simulink model "Model_with_decision_and_sieve"  (R2022a)
settings: Solver=VariableStepAuto  StartTime=0.0  StopTime=1000000  RelTol=1e-3
undefined symbols (not defined in the file): Coefficient_value, Enable_X, Enable_Y, N, s1, s10, s11, s12, s13, s14, s15, s16, s17, s18, s19, s2, s20, s21, s22, s23, s24, s25, s26, s27, s28, s29, s3, s30, s4, s5, s6, s7, s8, s9
libraries: simulink x37, dspsigops x2
(part 4 of 5)

== system Model_with_decision_and_sieve/Y12 ==
  Y1 : Inport  OutDataTypeStr=fixdt(0,1,0)  LockScale=on
  Y2 : Inport  Port=2  OutDataTypeStr=fixdt(0,1,0)  LockScale=on
  Y3 : Inport  Port=3  OutDataTypeStr=fixdt(0,1,0)  LockScale=on
  Y4 : Inport  Port=4  OutDataTypeStr=fixdt(0,1,0)  LockScale=on
  Y5 : Inport  Port=5  OutDataTypeStr=fixdt(0,1,0)  LockScale=on
  Y6 : Inport  Port=6  OutDataTypeStr=fixdt(0,1,0)  LockScale=on
  Y7 : Inport  Port=7  OutDataTypeStr=fixdt(0,1,0)  LockScale=on
  Y8 : Inport  Port=8  OutDataTypeStr=fixdt(0,1,0)  LockScale=on
  Y9 : Inport  Port=9  OutDataTypeStr=fixdt(0,1,0)  LockScale=on
  Y10 : Inport  Port=10  OutDataTypeStr=fixdt(0,1,0)  LockScale=on
  Y11 : Inport  Port=11  OutDataTypeStr=fixdt(0,1,0)  LockScale=on
  Y12 : Inport  Port=12  OutDataTypeStr=fixdt(0,1,0)  LockScale=on
  Y13 : Inport  Port=13  OutDataTypeStr=fixdt(0,1,0)  LockScale=on
  Y14 : Inport  Port=14  OutDataTypeStr=fixdt(0,1,0)  LockScale=on
  Y15 : Inport  Port=15  OutDataTypeStr=fixdt(0,1,0)  LockScale=on
  X : Inport  Port=16
  N : Inport  Port=17  LockScale=on
  shifted_coeff : Inport  Port=18  LockScale=on
  EN_Y : Inport  Port=19  OutDataTypeStr=fixdt(0,1,0)  LockScale=on
  Add : Sum  Inputs=++++++++++++++++
  Add2 : Sum  Inputs=+-
  Constant : Constant  Value=2
  Constant1 : Constant  Value=4
  Constant15 : Constant  Value=128
  Constant16 : Constant  Value=256
  Constant17 : Constant  Value=512
  Constant18 : Constant  Value=1024
  Constant19 : Constant  Value=2048
  Constant2 : Constant  Value=8
  Constant20 : Constant  Value=4096
  Constant21 : Constant  Value=8192
  Constant22 : Constant  Value=16384
  Constant3 : Constant  Value=16
  Constant34 : Constant  Value=32768
  Constant4 : Constant  Value=32
  Constant6 : Constant
  Constant8 : Constant  Value=64
  NOT : Logic  Operator=NOT  IconShape=distinctive  AllPortsSameDT=off  OutDataTypeStr=boolean
  Product{,1..6,8,16..23,35,142} (18 alike) : Product
  Switch_2 : Switch  Criteria=u2 ~= 0  OutDataTypeStr=fixdt(0,1,0)  SaturateOnIntegerOverflow=off  InputSameDT=off
  E_Y : Outport  LockScale=on
  wires:
  Constant/1 -> Product/2
  Y1/1 -> Product/1
  Constant1/1 -> Product1/2
  Y2/1 -> Product1/1
  Constant2/1 -> Product2/2
  Y3/1 -> Product2/1
  Constant6/1 -> Add/1
  Product/1 -> Add/2
  Product1/1 -> Add/3
  Product2/1 -> Add/4
  Add/1 -> Product6/1
  Add2/1 -> Product8/2, Product8/1
  Product4/1 -> Add/6
  Constant4/1 -> Product4/2
  Constant8/1 -> Product5/2
  Y6/1 -> Product5/1
  Product3/1 -> Add/5
  Y4/1 -> Product3/1
  Product5/1 -> Add/7
  Y5/1 -> Product4/1
  Constant3/1 -> Product3/2
  Product19/1 -> Add/11
  Constant20/1 -> Product21/2
  Constant18/1 -> Product19/2
  Product18/1 -> Add/10
  Constant15/1 -> Product16/2
  Constant16/1 -> Product17/2
  Y11/1 -> Product20/1
  Product20/1 -> Add/12
  Y8/1 -> Product17/1
  Y10/1 -> Product19/1
  Y7/1 -> Product16/1
  Constant19/1 -> Product20/2
  Product16/1 -> Add/8
  Y9/1 -> Product18/1
  Constant17/1 -> Product18/2
  Product21/1 -> Add/13
  Switch_2/1 -> Product21/1
  Product17/1 -> Add/9
  Y14/1 -> Product23/1
  Product22/1 -> Add/14
  Product23/1 -> Add/15
  Constant21/1 -> Product22/2
  Constant22/1 -> Product23/2
  [EN_Y] -> Switch_2/2
  Y12/1 -> Switch_2/3, NOT/1  "PBIT28"
  NOT/1 -> Switch_2/1
  Y13/1 -> Product22/1
  EN_Y/1 -> [EN_Y]
  shifted_coeff/1 -> [shifted_coeff]
  Product142/1 -> E_Y/1
  [shifted_coeff] -> Product142/2
  Product6/1 -> Add2/1
  Product8/1 -> Product142/1
  N/1 -> Add2/2
  X/1 -> Product6/2
  Y15/1 -> Product35/1
  Product35/1 -> Add/16
  Constant34/1 -> Product35/2

== system Model_with_decision_and_sieve/Y13 ==
  Y1 : Inport  OutDataTypeStr=fixdt(0,1,0)  LockScale=on
  Y2 : Inport  Port=2  OutDataTypeStr=fixdt(0,1,0)  LockScale=on
  Y3 : Inport  Port=3  OutDataTypeStr=fixdt(0,1,0)  LockScale=on
  Y4 : Inport  Port=4  OutDataTypeStr=fixdt(0,1,0)  LockScale=on
  Y5 : Inport  Port=5  OutDataTypeStr=fixdt(0,1,0)  LockScale=on
  Y6 : Inport  Port=6  OutDataTypeStr=fixdt(0,1,0)  LockScale=on
  Y7 : Inport  Port=7  OutDataTypeStr=fixdt(0,1,0)  LockScale=on
  Y8 : Inport  Port=8  OutDataTypeStr=fixdt(0,1,0)  LockScale=on
  Y9 : Inport  Port=9  OutDataTypeStr=fixdt(0,1,0)  LockScale=on
  Y10 : Inport  Port=10  OutDataTypeStr=fixdt(0,1,0)  LockScale=on
  Y11 : Inport  Port=11  OutDataTypeStr=fixdt(0,1,0)  LockScale=on
  Y12 : Inport  Port=12  OutDataTypeStr=fixdt(0,1,0)  LockScale=on
  Y13 : Inport  Port=13  OutDataTypeStr=fixdt(0,1,0)  LockScale=on
  Y14 : Inport  Port=14  OutDataTypeStr=fixdt(0,1,0)  LockScale=on
  Y15 : Inport  Port=15  OutDataTypeStr=fixdt(0,1,0)  LockScale=on
  X : Inport  Port=16
  N : Inport  Port=17  LockScale=on
  shifted_coeff : Inport  Port=18  LockScale=on
  EN_Y : Inport  Port=19  OutDataTypeStr=fixdt(0,1,0)  LockScale=on
  Add : Sum  Inputs=++++++++++++++++
  Add2 : Sum  Inputs=+-
  Constant : Constant  Value=2
  Constant1 : Constant  Value=4
  Constant15 : Constant  Value=128
  Constant16 : Constant  Value=256
  Constant17 : Constant  Value=512
  Constant18 : Constant  Value=1024
  Constant19 : Constant  Value=2048
  Constant2 : Constant  Value=8
  Constant20 : Constant  Value=4096
  Constant21 : Constant  Value=8192
  Constant22 : Constant  Value=16384
  Constant3 : Constant  Value=16
  Constant34 : Constant  Value=32768
  Constant4 : Constant  Value=32
  Constant6 : Constant
  Constant8 : Constant  Value=64
  NOT : Logic  Operator=NOT  IconShape=distinctive  AllPortsSameDT=off  OutDataTypeStr=boolean
  Product{,1..6,8,16..23,35,142} (18 alike) : Product
  Switch_2 : Switch  Criteria=u2 ~= 0  OutDataTypeStr=fixdt(0,1,0)  SaturateOnIntegerOverflow=off  InputSameDT=off
  E_Y : Outport  LockScale=on
  wires:
  Constant34/1 -> Product35/2
  Product35/1 -> Add/16
  Y15/1 -> Product35/1
  X/1 -> Product6/2
  N/1 -> Add2/2
  Product8/1 -> Product142/1
  Product6/1 -> Add2/1
  [shifted_coeff] -> Product142/2
  Product142/1 -> E_Y/1
  shifted_coeff/1 -> [shifted_coeff]
  EN_Y/1 -> [EN_Y]
  Switch_2/1 -> Product22/1
  NOT/1 -> Switch_2/1
  Y13/1 -> Switch_2/3, NOT/1  "PBIT28"
  [EN_Y] -> Switch_2/2
  Constant22/1 -> Product23/2
  Constant21/1 -> Product22/2
  Product23/1 -> Add/15
  Product22/1 -> Add/14
  Y14/1 -> Product23/1
  Product17/1 -> Add/9
  Y12/1 -> Product21/1
  Product21/1 -> Add/13
  Constant17/1 -> Product18/2
  Y9/1 -> Product18/1
  Product16/1 -> Add/8
  Constant19/1 -> Product20/2
  Y7/1 -> Product16/1
  Y10/1 -> Product19/1
  Y8/1 -> Product17/1
  Product20/1 -> Add/12
  Y11/1 -> Product20/1
  Constant16/1 -> Product17/2
  Constant15/1 -> Product16/2
  Product18/1 -> Add/10
  Constant18/1 -> Product19/2
  Constant20/1 -> Product21/2
  Product19/1 -> Add/11
  Constant3/1 -> Product3/2
  Y5/1 -> Product4/1
  Product5/1 -> Add/7
  Y4/1 -> Product3/1
  Product3/1 -> Add/5
  Y6/1 -> Product5/1
  Constant8/1 -> Product5/2
  Constant4/1 -> Product4/2
  Product4/1 -> Add/6
  Add2/1 -> Product8/1, Product8/2
  Add/1 -> Product6/1
  Product2/1 -> Add/4
  Product1/1 -> Add/3
  Product/1 -> Add/2
  Constant6/1 -> Add/1
  Y3/1 -> Product2/1
  Constant2/1 -> Product2/2
  Y2/1 -> Product1/1
  Constant1/1 -> Product1/2
  Y1/1 -> Product/1
  Constant/1 -> Product/2

== system Model_with_decision_and_sieve/Y14 ==
  Y1 : Inport  OutDataTypeStr=fixdt(0,1,0)  LockScale=on
  Y2 : Inport  Port=2  OutDataTypeStr=fixdt(0,1,0)  LockScale=on
  Y3 : Inport  Port=3  OutDataTypeStr=fixdt(0,1,0)  LockScale=on
  Y4 : Inport  Port=4  OutDataTypeStr=fixdt(0,1,0)  LockScale=on
  Y5 : Inport  Port=5  OutDataTypeStr=fixdt(0,1,0)  LockScale=on
  Y6 : Inport  Port=6  OutDataTypeStr=fixdt(0,1,0)  LockScale=on
  Y7 : Inport  Port=7  OutDataTypeStr=fixdt(0,1,0)  LockScale=on
  Y8 : Inport  Port=8  OutDataTypeStr=fixdt(0,1,0)  LockScale=on
  Y9 : Inport  Port=9  OutDataTypeStr=fixdt(0,1,0)  LockScale=on
  Y10 : Inport  Port=10  OutDataTypeStr=fixdt(0,1,0)  LockScale=on
  Y11 : Inport  Port=11  OutDataTypeStr=fixdt(0,1,0)  LockScale=on
  Y12 : Inport  Port=12  OutDataTypeStr=fixdt(0,1,0)  LockScale=on
  Y13 : Inport  Port=13  OutDataTypeStr=fixdt(0,1,0)  LockScale=on
  Y14 : Inport  Port=14  OutDataTypeStr=fixdt(0,1,0)  LockScale=on
  Y15 : Inport  Port=15  OutDataTypeStr=fixdt(0,1,0)  LockScale=on
  X : Inport  Port=16
  N : Inport  Port=17  LockScale=on
  shifted_coeff : Inport  Port=18  LockScale=on
  EN_Y : Inport  Port=19  OutDataTypeStr=fixdt(0,1,0)  LockScale=on
  Add : Sum  Inputs=++++++++++++++++
  Add2 : Sum  Inputs=+-
  Constant : Constant  Value=2
  Constant1 : Constant  Value=4
  Constant15 : Constant  Value=128
  Constant16 : Constant  Value=256
  Constant17 : Constant  Value=512
  Constant18 : Constant  Value=1024
  Constant19 : Constant  Value=2048
  Constant2 : Constant  Value=8
  Constant20 : Constant  Value=4096
  Constant21 : Constant  Value=8192
  Constant22 : Constant  Value=16384
  Constant3 : Constant  Value=16
  Constant34 : Constant  Value=32768
  Constant4 : Constant  Value=32
  Constant6 : Constant
  Constant8 : Constant  Value=64
  NOT : Logic  Operator=NOT  IconShape=distinctive  AllPortsSameDT=off  OutDataTypeStr=boolean
  Product{,1..6,8,16..23,35,142} (18 alike) : Product
  Switch_2 : Switch  Criteria=u2 ~= 0  OutDataTypeStr=fixdt(0,1,0)  SaturateOnIntegerOverflow=off  InputSameDT=off
  E_Y : Outport  LockScale=on
  wires:
  Constant/1 -> Product/2
  Y1/1 -> Product/1
  Constant1/1 -> Product1/2
  Y2/1 -> Product1/1
  Constant2/1 -> Product2/2
  Y3/1 -> Product2/1
  Constant6/1 -> Add/1
  Product/1 -> Add/2
  Product1/1 -> Add/3
  Product2/1 -> Add/4
  Add/1 -> Product6/1
  Add2/1 -> Product8/2, Product8/1
  Product4/1 -> Add/6
  Constant4/1 -> Product4/2
  Constant8/1 -> Product5/2
  Y6/1 -> Product5/1
  Product3/1 -> Add/5
  Y4/1 -> Product3/1
  Product5/1 -> Add/7
  Y5/1 -> Product4/1
  Constant3/1 -> Product3/2
  Product19/1 -> Add/11
  Constant20/1 -> Product21/2
  Constant18/1 -> Product19/2
  Product18/1 -> Add/10
  Constant15/1 -> Product16/2
  Constant16/1 -> Product17/2
  Y11/1 -> Product20/1
  Product20/1 -> Add/12
  Y8/1 -> Product17/1
  Y10/1 -> Product19/1
  Y7/1 -> Product16/1
  Constant19/1 -> Product20/2
  Product16/1 -> Add/8
  Y9/1 -> Product18/1
  Constant17/1 -> Product18/2
  Product21/1 -> Add/13
  Y12/1 -> Product21/1
  Product17/1 -> Add/9
  Switch_2/1 -> Product23/1
  Product22/1 -> Add/14
  Product23/1 -> Add/15
  Constant21/1 -> Product22/2
  Constant22/1 -> Product23/2
  [EN_Y] -> Switch_2/2
  Y14/1 -> Switch_2/3, NOT/1  "PBIT28"
  NOT/1 -> Switch_2/1
  Y13/1 -> Product22/1
  EN_Y/1 -> [EN_Y]
  shifted_coeff/1 -> [shifted_coeff]
  Product142/1 -> E_Y/1
  [shifted_coeff] -> Product142/2
  Product6/1 -> Add2/1
  Product8/1 -> Product142/1
  N/1 -> Add2/2
  X/1 -> Product6/2
  Y15/1 -> Product35/1
  Product35/1 -> Add/16
  Constant34/1 -> Product35/2

== system Model_with_decision_and_sieve/Y15 ==
  Y1 : Inport  OutDataTypeStr=fixdt(0,1,0)  LockScale=on
  Y2 : Inport  Port=2  OutDataTypeStr=fixdt(0,1,0)  LockScale=on
  Y3 : Inport  Port=3  OutDataTypeStr=fixdt(0,1,0)  LockScale=on
  Y4 : Inport  Port=4  OutDataTypeStr=fixdt(0,1,0)  LockScale=on
  Y5 : Inport  Port=5  OutDataTypeStr=fixdt(0,1,0)  LockScale=on
  Y6 : Inport  Port=6  OutDataTypeStr=fixdt(0,1,0)  LockScale=on
  Y7 : Inport  Port=7  OutDataTypeStr=fixdt(0,1,0)  LockScale=on
  Y8 : Inport  Port=8  OutDataTypeStr=fixdt(0,1,0)  LockScale=on
  Y9 : Inport  Port=9  OutDataTypeStr=fixdt(0,1,0)  LockScale=on
  Y10 : Inport  Port=10  OutDataTypeStr=fixdt(0,1,0)  LockScale=on
  Y11 : Inport  Port=11  OutDataTypeStr=fixdt(0,1,0)  LockScale=on
  Y12 : Inport  Port=12  OutDataTypeStr=fixdt(0,1,0)  LockScale=on
  Y13 : Inport  Port=13  OutDataTypeStr=fixdt(0,1,0)  LockScale=on
  Y14 : Inport  Port=14  OutDataTypeStr=fixdt(0,1,0)  LockScale=on
  Y15 : Inport  Port=15  OutDataTypeStr=fixdt(0,1,0)  LockScale=on
  X : Inport  Port=16
  N : Inport  Port=17  LockScale=on
  shifted_coeff : Inport  Port=18  LockScale=on
  EN_Y : Inport  Port=19  OutDataTypeStr=fixdt(0,1,0)  LockScale=on
  Add : Sum  Inputs=++++++++++++++++
  Add2 : Sum  Inputs=+-
  Constant : Constant  Value=2
  Constant1 : Constant  Value=4
  Constant15 : Constant  Value=128
  Constant16 : Constant  Value=256
  Constant17 : Constant  Value=512
  Constant18 : Constant  Value=1024
  Constant19 : Constant  Value=2048
  Constant2 : Constant  Value=8
  Constant20 : Constant  Value=4096
  Constant21 : Constant  Value=8192
  Constant22 : Constant  Value=16384
  Constant3 : Constant  Value=16
  Constant34 : Constant  Value=32768
  Constant4 : Constant  Value=32
  Constant6 : Constant
  Constant8 : Constant  Value=64
  NOT : Logic  Operator=NOT  IconShape=distinctive  AllPortsSameDT=off  OutDataTypeStr=boolean
  Product{,1..6,8,16..23,35,142} (18 alike) : Product
  Switch_2 : Switch  Criteria=u2 ~= 0  OutDataTypeStr=fixdt(0,1,0)  SaturateOnIntegerOverflow=off  InputSameDT=off
  E_Y : Outport  LockScale=on
  wires:
  Constant34/1 -> Product35/2
  Product35/1 -> Add/16
  Switch_2/1 -> Product35/1
  X/1 -> Product6/2
  N/1 -> Add2/2
  Product8/1 -> Product142/1
  Product6/1 -> Add2/1
  [shifted_coeff] -> Product142/2
  Product142/1 -> E_Y/1
  shifted_coeff/1 -> [shifted_coeff]
  EN_Y/1 -> [EN_Y]
  Y13/1 -> Product22/1
  NOT/1 -> Switch_2/1
  Y15/1 -> NOT/1, Switch_2/3  "PBIT28"
  [EN_Y] -> Switch_2/2
  Constant22/1 -> Product23/2
  Constant21/1 -> Product22/2
  Product23/1 -> Add/15
  Product22/1 -> Add/14
  Y14/1 -> Product23/1
  Product17/1 -> Add/9
  Y12/1 -> Product21/1
  Product21/1 -> Add/13
  Constant17/1 -> Product18/2
  Y9/1 -> Product18/1
  Product16/1 -> Add/8
  Constant19/1 -> Product20/2
  Y7/1 -> Product16/1
  Y10/1 -> Product19/1
  Y8/1 -> Product17/1
  Product20/1 -> Add/12
  Y11/1 -> Product20/1
  Constant16/1 -> Product17/2
  Constant15/1 -> Product16/2
  Product18/1 -> Add/10
  Constant18/1 -> Product19/2
  Constant20/1 -> Product21/2
  Product19/1 -> Add/11
  Constant3/1 -> Product3/2
  Y5/1 -> Product4/1
  Product5/1 -> Add/7
  Y4/1 -> Product3/1
  Product3/1 -> Add/5
  Y6/1 -> Product5/1
  Constant8/1 -> Product5/2
  Constant4/1 -> Product4/2
  Product4/1 -> Add/6
  Add2/1 -> Product8/1, Product8/2
  Add/1 -> Product6/1
  Product2/1 -> Add/4
  Product1/1 -> Add/3
  Product/1 -> Add/2
  Constant6/1 -> Add/1
  Y3/1 -> Product2/1
  Constant2/1 -> Product2/2
  Y2/1 -> Product1/1
  Constant1/1 -> Product1/2
  Y1/1 -> Product/1
  Constant/1 -> Product/2

== system Model_with_decision_and_sieve/Y2 ==
  Y1 : Inport  OutDataTypeStr=fixdt(0,1,0)  LockScale=on
  Y2 : Inport  Port=2  OutDataTypeStr=fixdt(0,1,0)  LockScale=on
  Y3 : Inport  Port=3  OutDataTypeStr=fixdt(0,1,0)  LockScale=on
  Y4 : Inport  Port=4  OutDataTypeStr=fixdt(0,1,0)  LockScale=on
  Y5 : Inport  Port=5  OutDataTypeStr=fixdt(0,1,0)  LockScale=on
  Y6 : Inport  Port=6  OutDataTypeStr=fixdt(0,1,0)  LockScale=on
  Y7 : Inport  Port=7  OutDataTypeStr=fixdt(0,1,0)  LockScale=on
  Y8 : Inport  Port=8  OutDataTypeStr=fixdt(0,1,0)  LockScale=on
  Y9 : Inport  Port=9  OutDataTypeStr=fixdt(0,1,0)  LockScale=on
  Y10 : Inport  Port=10  OutDataTypeStr=fixdt(0,1,0)  LockScale=on
  Y11 : Inport  Port=11  OutDataTypeStr=fixdt(0,1,0)  LockScale=on
  Y12 : Inport  Port=12  OutDataTypeStr=fixdt(0,1,0)  LockScale=on
  Y13 : Inport  Port=13  OutDataTypeStr=fixdt(0,1,0)  LockScale=on
  Y14 : Inport  Port=14  OutDataTypeStr=fixdt(0,1,0)  LockScale=on
  Y15 : Inport  Port=15  OutDataTypeStr=fixdt(0,1,0)  LockScale=on
  X : Inport  Port=16
  N : Inport  Port=17  LockScale=on
  shifted_coeff : Inport  Port=18  LockScale=on
  EN_Y : Inport  Port=19  OutDataTypeStr=fixdt(0,1,0)  LockScale=on
  Add : Sum  Inputs=++++++++++++++++
  Add2 : Sum  Inputs=+-
  Constant : Constant  Value=2
  Constant1 : Constant  Value=4
  Constant15 : Constant  Value=128
  Constant16 : Constant  Value=256
  Constant17 : Constant  Value=512
  Constant18 : Constant  Value=1024
  Constant19 : Constant  Value=2048
  Constant2 : Constant  Value=8
  Constant20 : Constant  Value=4096
  Constant21 : Constant  Value=8192
  Constant22 : Constant  Value=16384
  Constant3 : Constant  Value=16
  Constant34 : Constant  Value=32768
  Constant4 : Constant  Value=32
  Constant6 : Constant
  Constant8 : Constant  Value=64
  NOT : Logic  Operator=NOT  IconShape=distinctive  AllPortsSameDT=off  OutDataTypeStr=boolean
  Product{,1..6,8,16..23,35,142} (18 alike) : Product
  Switch_2 : Switch  Criteria=u2 ~= 0  OutDataTypeStr=fixdt(0,1,0)  SaturateOnIntegerOverflow=off  InputSameDT=off
  E_Y : Outport  LockScale=on
  wires:
  Constant34/1 -> Product35/2
  Product35/1 -> Add/16
  Y15/1 -> Product35/1
  X/1 -> Product6/2
  N/1 -> Add2/2
  Product8/1 -> Product142/1
  Product6/1 -> Add2/1
  [shifted_coeff] -> Product142/2
  Product142/1 -> E_Y/1
  shifted_coeff/1 -> [shifted_coeff]
  EN_Y/1 -> [EN_Y]
  Y13/1 -> Product22/1
  NOT/1 -> Switch_2/1
  Y2/1 -> Switch_2/3, NOT/1  "PBIT28"
  [EN_Y] -> Switch_2/2
  Constant22/1 -> Product23/2
  Constant21/1 -> Product22/2
  Product23/1 -> Add/15
  Product22/1 -> Add/14
  Y14/1 -> Product23/1
  Product17/1 -> Add/9
  Y12/1 -> Product21/1
  Product21/1 -> Add/13
  Constant17/1 -> Product18/2
  Y9/1 -> Product18/1
  Product16/1 -> Add/8
  Constant19/1 -> Product20/2
  Y7/1 -> Product16/1
  Y10/1 -> Product19/1
  Y8/1 -> Product17/1
  Product20/1 -> Add/12
  Y11/1 -> Product20/1
  Constant16/1 -> Product17/2
  Constant15/1 -> Product16/2
  Product18/1 -> Add/10
  Constant18/1 -> Product19/2
  Constant20/1 -> Product21/2
  Product19/1 -> Add/11
  Constant3/1 -> Product3/2
  Y5/1 -> Product4/1
  Product5/1 -> Add/7
  Y4/1 -> Product3/1
  Product3/1 -> Add/5
  Y6/1 -> Product5/1
  Constant8/1 -> Product5/2
  Constant4/1 -> Product4/2
  Product4/1 -> Add/6
  Add2/1 -> Product8/1, Product8/2
  Add/1 -> Product6/1
  Product2/1 -> Add/4
  Product1/1 -> Add/3
  Product/1 -> Add/2
  Constant6/1 -> Add/1
  Y3/1 -> Product2/1
  Constant2/1 -> Product2/2
  Switch_2/1 -> Product1/1
  Constant1/1 -> Product1/2
  Y1/1 -> Product/1
  Constant/1 -> Product/2

== system Model_with_decision_and_sieve/Y3 ==
  Y1 : Inport  OutDataTypeStr=fixdt(0,1,0)  LockScale=on
  Y2 : Inport  Port=2  OutDataTypeStr=fixdt(0,1,0)  LockScale=on
  Y3 : Inport  Port=3  OutDataTypeStr=fixdt(0,1,0)  LockScale=on
  Y4 : Inport  Port=4  OutDataTypeStr=fixdt(0,1,0)  LockScale=on
  Y5 : Inport  Port=5  OutDataTypeStr=fixdt(0,1,0)  LockScale=on
  Y6 : Inport  Port=6  OutDataTypeStr=fixdt(0,1,0)  LockScale=on
  Y7 : Inport  Port=7  OutDataTypeStr=fixdt(0,1,0)  LockScale=on
  Y8 : Inport  Port=8  OutDataTypeStr=fixdt(0,1,0)  LockScale=on
  Y9 : Inport  Port=9  OutDataTypeStr=fixdt(0,1,0)  LockScale=on
  Y10 : Inport  Port=10  OutDataTypeStr=fixdt(0,1,0)  LockScale=on
  Y11 : Inport  Port=11  OutDataTypeStr=fixdt(0,1,0)  LockScale=on
  Y12 : Inport  Port=12  OutDataTypeStr=fixdt(0,1,0)  LockScale=on
  Y13 : Inport  Port=13  OutDataTypeStr=fixdt(0,1,0)  LockScale=on
  Y14 : Inport  Port=14  OutDataTypeStr=fixdt(0,1,0)  LockScale=on
  Y15 : Inport  Port=15  OutDataTypeStr=fixdt(0,1,0)  LockScale=on
  X : Inport  Port=16
  N : Inport  Port=17  LockScale=on
  shifted_coeff : Inport  Port=18  LockScale=on
  EN_Y : Inport  Port=19  OutDataTypeStr=fixdt(0,1,0)  LockScale=on
  Add : Sum  Inputs=++++++++++++++++
  Add2 : Sum  Inputs=+-
  Constant : Constant  Value=2
  Constant1 : Constant  Value=4
  Constant15 : Constant  Value=128
  Constant16 : Constant  Value=256
  Constant17 : Constant  Value=512
  Constant18 : Constant  Value=1024
  Constant19 : Constant  Value=2048
  Constant2 : Constant  Value=8
  Constant20 : Constant  Value=4096
  Constant21 : Constant  Value=8192
  Constant22 : Constant  Value=16384
  Constant3 : Constant  Value=16
  Constant34 : Constant  Value=32768
  Constant4 : Constant  Value=32
  Constant6 : Constant
  Constant8 : Constant  Value=64
  NOT : Logic  Operator=NOT  IconShape=distinctive  AllPortsSameDT=off  OutDataTypeStr=boolean
  Product{,1..6,8,16..23,35,142} (18 alike) : Product
  Switch_2 : Switch  Criteria=u2 ~= 0  OutDataTypeStr=fixdt(0,1,0)  SaturateOnIntegerOverflow=off  InputSameDT=off
  E_Y : Outport  LockScale=on
  wires:
  Constant/1 -> Product/2
  Y1/1 -> Product/1
  Constant1/1 -> Product1/2
  Y2/1 -> Product1/1
  Constant2/1 -> Product2/2
  Switch_2/1 -> Product2/1
  Constant6/1 -> Add/1
  Product/1 -> Add/2
  Product1/1 -> Add/3
  Product2/1 -> Add/4
  Add/1 -> Product6/1
  Add2/1 -> Product8/2, Product8/1
  Product4/1 -> Add/6
  Constant4/1 -> Product4/2
  Constant8/1 -> Product5/2
  Y6/1 -> Product5/1
  Product3/1 -> Add/5
  Y4/1 -> Product3/1
  Product5/1 -> Add/7
  Y5/1 -> Product4/1
  Constant3/1 -> Product3/2
  Product19/1 -> Add/11
  Constant20/1 -> Product21/2
  Constant18/1 -> Product19/2
  Product18/1 -> Add/10
  Constant15/1 -> Product16/2
  Constant16/1 -> Product17/2
  Y11/1 -> Product20/1
  Product20/1 -> Add/12
  Y8/1 -> Product17/1
  Y10/1 -> Product19/1
  Y7/1 -> Product16/1
  Constant19/1 -> Product20/2
  Product16/1 -> Add/8
  Y9/1 -> Product18/1
  Constant17/1 -> Product18/2
  Product21/1 -> Add/13
  Y12/1 -> Product21/1
  Product17/1 -> Add/9
  Y14/1 -> Product23/1
  Product22/1 -> Add/14
  Product23/1 -> Add/15
  Constant21/1 -> Product22/2
  Constant22/1 -> Product23/2
  [EN_Y] -> Switch_2/2
  Y3/1 -> NOT/1, Switch_2/3  "PBIT28"
  NOT/1 -> Switch_2/1
  Y13/1 -> Product22/1
  EN_Y/1 -> [EN_Y]
  shifted_coeff/1 -> [shifted_coeff]
  Product142/1 -> E_Y/1
  [shifted_coeff] -> Product142/2
  Product6/1 -> Add2/1
  Product8/1 -> Product142/1
  N/1 -> Add2/2
  X/1 -> Product6/2
  Y15/1 -> Product35/1
  Product35/1 -> Add/16
  Constant34/1 -> Product35/2

== system Model_with_decision_and_sieve/Y4 ==
  Y1 : Inport  OutDataTypeStr=fixdt(0,1,0)  LockScale=on
  Y2 : Inport  Port=2  OutDataTypeStr=fixdt(0,1,0)  LockScale=on
  Y3 : Inport  Port=3  OutDataTypeStr=fixdt(0,1,0)  LockScale=on
  Y4 : Inport  Port=4  OutDataTypeStr=fixdt(0,1,0)  LockScale=on
  Y5 : Inport  Port=5  OutDataTypeStr=fixdt(0,1,0)  LockScale=on
  Y6 : Inport  Port=6  OutDataTypeStr=fixdt(0,1,0)  LockScale=on
  Y7 : Inport  Port=7  OutDataTypeStr=fixdt(0,1,0)  LockScale=on
  Y8 : Inport  Port=8  OutDataTypeStr=fixdt(0,1,0)  LockScale=on
  Y9 : Inport  Port=9  OutDataTypeStr=fixdt(0,1,0)  LockScale=on
  Y10 : Inport  Port=10  OutDataTypeStr=fixdt(0,1,0)  LockScale=on
  Y11 : Inport  Port=11  OutDataTypeStr=fixdt(0,1,0)  LockScale=on
  Y12 : Inport  Port=12  OutDataTypeStr=fixdt(0,1,0)  LockScale=on
  Y13 : Inport  Port=13  OutDataTypeStr=fixdt(0,1,0)  LockScale=on
  Y14 : Inport  Port=14  OutDataTypeStr=fixdt(0,1,0)  LockScale=on
  Y15 : Inport  Port=15  OutDataTypeStr=fixdt(0,1,0)  LockScale=on
  X : Inport  Port=16
  N : Inport  Port=17  LockScale=on
  shifted_coeff : Inport  Port=18  LockScale=on
  EN_Y : Inport  Port=19  OutDataTypeStr=fixdt(0,1,0)  LockScale=on
  Add : Sum  Inputs=++++++++++++++++
  Add2 : Sum  Inputs=+-
  Constant : Constant  Value=2
  Constant1 : Constant  Value=4
  Constant15 : Constant  Value=128
  Constant16 : Constant  Value=256
  Constant17 : Constant  Value=512
  Constant18 : Constant  Value=1024
  Constant19 : Constant  Value=2048
  Constant2 : Constant  Value=8
  Constant20 : Constant  Value=4096
  Constant21 : Constant  Value=8192
  Constant22 : Constant  Value=16384
  Constant3 : Constant  Value=16
  Constant34 : Constant  Value=32768
  Constant4 : Constant  Value=32
  Constant6 : Constant
  Constant8 : Constant  Value=64
  NOT : Logic  Operator=NOT  IconShape=distinctive  AllPortsSameDT=off  OutDataTypeStr=boolean
  Product{,1..6,8,16..23,35,142} (18 alike) : Product
  Switch_2 : Switch  Criteria=u2 ~= 0  OutDataTypeStr=fixdt(0,1,0)  SaturateOnIntegerOverflow=off  InputSameDT=off
  E_Y : Outport  LockScale=on
  wires:
  Constant34/1 -> Product35/2
  Product35/1 -> Add/16
  Y15/1 -> Product35/1
  X/1 -> Product6/2
  N/1 -> Add2/2
  Product8/1 -> Product142/1
  Product6/1 -> Add2/1
  [shifted_coeff] -> Product142/2
  Product142/1 -> E_Y/1
  shifted_coeff/1 -> [shifted_coeff]
  EN_Y/1 -> [EN_Y]
  Y13/1 -> Product22/1
  NOT/1 -> Switch_2/1
  Y4/1 -> Switch_2/3, NOT/1  "PBIT28"
  [EN_Y] -> Switch_2/2
  Constant22/1 -> Product23/2
  Constant21/1 -> Product22/2
  Product23/1 -> Add/15
  Product22/1 -> Add/14
  Y14/1 -> Product23/1
  Product17/1 -> Add/9
  Y12/1 -> Product21/1
  Product21/1 -> Add/13
  Constant17/1 -> Product18/2
  Y9/1 -> Product18/1
  Product16/1 -> Add/8
  Constant19/1 -> Product20/2
  Y7/1 -> Product16/1
  Y10/1 -> Product19/1
  Y8/1 -> Product17/1
  Product20/1 -> Add/12
  Y11/1 -> Product20/1
  Constant16/1 -> Product17/2
  Constant15/1 -> Product16/2
  Product18/1 -> Add/10
  Constant18/1 -> Product19/2
  Constant20/1 -> Product21/2
  Product19/1 -> Add/11
  Constant3/1 -> Product3/2
  Y5/1 -> Product4/1
  Product5/1 -> Add/7
  Switch_2/1 -> Product3/1
  Product3/1 -> Add/5
  Y6/1 -> Product5/1
  Constant8/1 -> Product5/2
  Constant4/1 -> Product4/2
  Product4/1 -> Add/6
  Add2/1 -> Product8/1, Product8/2
  Add/1 -> Product6/1
  Product2/1 -> Add/4
  Product1/1 -> Add/3
  Product/1 -> Add/2
  Constant6/1 -> Add/1
  Y3/1 -> Product2/1
  Constant2/1 -> Product2/2
  Y2/1 -> Product1/1
  Constant1/1 -> Product1/2
  Y1/1 -> Product/1
  Constant/1 -> Product/2

== system Model_with_decision_and_sieve/Y5 ==
  Y1 : Inport  OutDataTypeStr=fixdt(0,1,0)  LockScale=on
  Y2 : Inport  Port=2  OutDataTypeStr=fixdt(0,1,0)  LockScale=on
  Y3 : Inport  Port=3  OutDataTypeStr=fixdt(0,1,0)  LockScale=on
  Y4 : Inport  Port=4  OutDataTypeStr=fixdt(0,1,0)  LockScale=on
  Y5 : Inport  Port=5  OutDataTypeStr=fixdt(0,1,0)  LockScale=on
  Y6 : Inport  Port=6  OutDataTypeStr=fixdt(0,1,0)  LockScale=on
  Y7 : Inport  Port=7  OutDataTypeStr=fixdt(0,1,0)  LockScale=on
  Y8 : Inport  Port=8  OutDataTypeStr=fixdt(0,1,0)  LockScale=on
  Y9 : Inport  Port=9  OutDataTypeStr=fixdt(0,1,0)  LockScale=on
  Y10 : Inport  Port=10  OutDataTypeStr=fixdt(0,1,0)  LockScale=on
  Y11 : Inport  Port=11  OutDataTypeStr=fixdt(0,1,0)  LockScale=on
  Y12 : Inport  Port=12  OutDataTypeStr=fixdt(0,1,0)  LockScale=on
  Y13 : Inport  Port=13  OutDataTypeStr=fixdt(0,1,0)  LockScale=on
  Y14 : Inport  Port=14  OutDataTypeStr=fixdt(0,1,0)  LockScale=on
  Y15 : Inport  Port=15  OutDataTypeStr=fixdt(0,1,0)  LockScale=on
  X : Inport  Port=16
  N : Inport  Port=17  LockScale=on
  shifted_coeff : Inport  Port=18  LockScale=on
  EN_Y : Inport  Port=19  OutDataTypeStr=fixdt(0,1,0)  LockScale=on
  Add : Sum  Inputs=++++++++++++++++
  Add2 : Sum  Inputs=+-
  Constant : Constant  Value=2
  Constant1 : Constant  Value=4
  Constant15 : Constant  Value=128
  Constant16 : Constant  Value=256
  Constant17 : Constant  Value=512
  Constant18 : Constant  Value=1024
  Constant19 : Constant  Value=2048
  Constant2 : Constant  Value=8
  Constant20 : Constant  Value=4096
  Constant21 : Constant  Value=8192
  Constant22 : Constant  Value=16384
  Constant3 : Constant  Value=16
  Constant34 : Constant  Value=32768
  Constant4 : Constant  Value=32
  Constant6 : Constant
  Constant8 : Constant  Value=64
  NOT : Logic  Operator=NOT  IconShape=distinctive  AllPortsSameDT=off  OutDataTypeStr=boolean
  Product{,1..6,8,16..23,35,142} (18 alike) : Product
  Switch_2 : Switch  Criteria=u2 ~= 0  OutDataTypeStr=fixdt(0,1,0)  SaturateOnIntegerOverflow=off  InputSameDT=off
  E_Y : Outport  LockScale=on
  wires:
  Constant/1 -> Product/2
  Y1/1 -> Product/1
  Constant1/1 -> Product1/2
  Y2/1 -> Product1/1
  Constant2/1 -> Product2/2
  Y3/1 -> Product2/1
  Constant6/1 -> Add/1
  Product/1 -> Add/2
  Product1/1 -> Add/3
  Product2/1 -> Add/4
  Add/1 -> Product6/1
  Add2/1 -> Product8/2, Product8/1
  Product4/1 -> Add/6
  Constant4/1 -> Product4/2
  Constant8/1 -> Product5/2
  Y6/1 -> Product5/1
  Product3/1 -> Add/5
  Y4/1 -> Product3/1
  Product5/1 -> Add/7
  Switch_2/1 -> Product4/1
  Constant3/1 -> Product3/2
  Product19/1 -> Add/11
  Constant20/1 -> Product21/2
  Constant18/1 -> Product19/2
  Product18/1 -> Add/10
  Constant15/1 -> Product16/2
  Constant16/1 -> Product17/2
  Y11/1 -> Product20/1
  Product20/1 -> Add/12
  Y8/1 -> Product17/1
  Y10/1 -> Product19/1
  Y7/1 -> Product16/1
  Constant19/1 -> Product20/2
  Product16/1 -> Add/8
  Y9/1 -> Product18/1
  Constant17/1 -> Product18/2
  Product21/1 -> Add/13
  Y12/1 -> Product21/1
  Product17/1 -> Add/9
  Y14/1 -> Product23/1
  Product22/1 -> Add/14
  Product23/1 -> Add/15
  Constant21/1 -> Product22/2
  Constant22/1 -> Product23/2
  [EN_Y] -> Switch_2/2
  Y5/1 -> NOT/1, Switch_2/3  "PBIT28"
  NOT/1 -> Switch_2/1
  Y13/1 -> Product22/1
  EN_Y/1 -> [EN_Y]
  shifted_coeff/1 -> [shifted_coeff]
  Product142/1 -> E_Y/1
  [shifted_coeff] -> Product142/2
  Product6/1 -> Add2/1
  Product8/1 -> Product142/1
  N/1 -> Add2/2
  X/1 -> Product6/2
  Y15/1 -> Product35/1
  Product35/1 -> Add/16
  Constant34/1 -> Product35/2

== system Model_with_decision_and_sieve/Y6 ==
  Y1 : Inport  OutDataTypeStr=fixdt(0,1,0)  LockScale=on
  Y2 : Inport  Port=2  OutDataTypeStr=fixdt(0,1,0)  LockScale=on
  Y3 : Inport  Port=3  OutDataTypeStr=fixdt(0,1,0)  LockScale=on
  Y4 : Inport  Port=4  OutDataTypeStr=fixdt(0,1,0)  LockScale=on
  Y5 : Inport  Port=5  OutDataTypeStr=fixdt(0,1,0)  LockScale=on
  Y6 : Inport  Port=6  OutDataTypeStr=fixdt(0,1,0)  LockScale=on
  Y7 : Inport  Port=7  OutDataTypeStr=fixdt(0,1,0)  LockScale=on
  Y8 : Inport  Port=8  OutDataTypeStr=fixdt(0,1,0)  LockScale=on
  Y9 : Inport  Port=9  OutDataTypeStr=fixdt(0,1,0)  LockScale=on
  Y10 : Inport  Port=10  OutDataTypeStr=fixdt(0,1,0)  LockScale=on
  Y11 : Inport  Port=11  OutDataTypeStr=fixdt(0,1,0)  LockScale=on
  Y12 : Inport  Port=12  OutDataTypeStr=fixdt(0,1,0)  LockScale=on
  Y13 : Inport  Port=13  OutDataTypeStr=fixdt(0,1,0)  LockScale=on
  Y14 : Inport  Port=14  OutDataTypeStr=fixdt(0,1,0)  LockScale=on
  Y15 : Inport  Port=15  OutDataTypeStr=fixdt(0,1,0)  LockScale=on
  X : Inport  Port=16
  N : Inport  Port=17  LockScale=on
  shifted_coeff : Inport  Port=18  LockScale=on
  EN_Y : Inport  Port=19  OutDataTypeStr=fixdt(0,1,0)  LockScale=on
  Add : Sum  Inputs=++++++++++++++++
  Add2 : Sum  Inputs=+-
  Constant : Constant  Value=2
  Constant1 : Constant  Value=4
  Constant15 : Constant  Value=128
  Constant16 : Constant  Value=256
  Constant17 : Constant  Value=512
  Constant18 : Constant  Value=1024
  Constant19 : Constant  Value=2048
  Constant2 : Constant  Value=8
  Constant20 : Constant  Value=4096
  Constant21 : Constant  Value=8192
  Constant22 : Constant  Value=16384
  Constant3 : Constant  Value=16
  Constant34 : Constant  Value=32768
  Constant4 : Constant  Value=32
  Constant6 : Constant
  Constant8 : Constant  Value=64
  NOT : Logic  Operator=NOT  IconShape=distinctive  AllPortsSameDT=off  OutDataTypeStr=boolean
  Product{,1..6,8,16..23,35,142} (18 alike) : Product
  Switch_2 : Switch  Criteria=u2 ~= 0  OutDataTypeStr=fixdt(0,1,0)  SaturateOnIntegerOverflow=off  InputSameDT=off
  E_Y : Outport  LockScale=on
  wires:
  Constant34/1 -> Product35/2
  Product35/1 -> Add/16
  Y15/1 -> Product35/1
  X/1 -> Product6/2
  N/1 -> Add2/2
  Product8/1 -> Product142/1
  Product6/1 -> Add2/1
  [shifted_coeff] -> Product142/2
  Product142/1 -> E_Y/1
  shifted_coeff/1 -> [shifted_coeff]
  EN_Y/1 -> [EN_Y]
  Y13/1 -> Product22/1
  NOT/1 -> Switch_2/1
  Y6/1 -> Switch_2/3, NOT/1  "PBIT28"
  [EN_Y] -> Switch_2/2
  Constant22/1 -> Product23/2
  Constant21/1 -> Product22/2
  Product23/1 -> Add/15
  Product22/1 -> Add/14
  Y14/1 -> Product23/1
  Product17/1 -> Add/9
  Y12/1 -> Product21/1
  Product21/1 -> Add/13
  Constant17/1 -> Product18/2
  Y9/1 -> Product18/1
  Product16/1 -> Add/8
  Constant19/1 -> Product20/2
  Y7/1 -> Product16/1
  Y10/1 -> Product19/1
  Y8/1 -> Product17/1
  Product20/1 -> Add/12
  Y11/1 -> Product20/1
  Constant16/1 -> Product17/2
  Constant15/1 -> Product16/2
  Product18/1 -> Add/10
  Constant18/1 -> Product19/2
  Constant20/1 -> Product21/2
  Product19/1 -> Add/11
  Constant3/1 -> Product3/2
  Y5/1 -> Product4/1
  Product5/1 -> Add/7
  Y4/1 -> Product3/1
  Product3/1 -> Add/5
  Switch_2/1 -> Product5/1
  Constant8/1 -> Product5/2
  Constant4/1 -> Product4/2
  Product4/1 -> Add/6
  Add2/1 -> Product8/1, Product8/2
  Add/1 -> Product6/1
  Product2/1 -> Add/4
  Product1/1 -> Add/3
  Product/1 -> Add/2
  Constant6/1 -> Add/1
  Y3/1 -> Product2/1
  Constant2/1 -> Product2/2
  Y2/1 -> Product1/1
  Constant1/1 -> Product1/2
  Y1/1 -> Product/1
  Constant/1 -> Product/2

== system Model_with_decision_and_sieve/Y7 ==
  Y1 : Inport  OutDataTypeStr=fixdt(0,1,0)  LockScale=on
  Y2 : Inport  Port=2  OutDataTypeStr=fixdt(0,1,0)  LockScale=on
  Y3 : Inport  Port=3  OutDataTypeStr=fixdt(0,1,0)  LockScale=on
  Y4 : Inport  Port=4  OutDataTypeStr=fixdt(0,1,0)  LockScale=on
  Y5 : Inport  Port=5  OutDataTypeStr=fixdt(0,1,0)  LockScale=on
  Y6 : Inport  Port=6  OutDataTypeStr=fixdt(0,1,0)  LockScale=on
  Y7 : Inport  Port=7  OutDataTypeStr=fixdt(0,1,0)  LockScale=on
  Y8 : Inport  Port=8  OutDataTypeStr=fixdt(0,1,0)  LockScale=on
  Y9 : Inport  Port=9  OutDataTypeStr=fixdt(0,1,0)  LockScale=on
  Y10 : Inport  Port=10  OutDataTypeStr=fixdt(0,1,0)  LockScale=on
  Y11 : Inport  Port=11  OutDataTypeStr=fixdt(0,1,0)  LockScale=on
  Y12 : Inport  Port=12  OutDataTypeStr=fixdt(0,1,0)  LockScale=on
  Y13 : Inport  Port=13  OutDataTypeStr=fixdt(0,1,0)  LockScale=on
  Y14 : Inport  Port=14  OutDataTypeStr=fixdt(0,1,0)  LockScale=on
  Y15 : Inport  Port=15  OutDataTypeStr=fixdt(0,1,0)  LockScale=on
  X : Inport  Port=16
  N : Inport  Port=17  LockScale=on
  shifted_coeff : Inport  Port=18  LockScale=on
  EN_Y : Inport  Port=19  OutDataTypeStr=fixdt(0,1,0)  LockScale=on
  Add : Sum  Inputs=++++++++++++++++
  Add2 : Sum  Inputs=+-
  Constant : Constant  Value=2
  Constant1 : Constant  Value=4
  Constant15 : Constant  Value=128
  Constant16 : Constant  Value=256
  Constant17 : Constant  Value=512
  Constant18 : Constant  Value=1024
  Constant19 : Constant  Value=2048
  Constant2 : Constant  Value=8
  Constant20 : Constant  Value=4096
  Constant21 : Constant  Value=8192
  Constant22 : Constant  Value=16384
  Constant3 : Constant  Value=16
  Constant34 : Constant  Value=32768
  Constant4 : Constant  Value=32
  Constant6 : Constant
  Constant8 : Constant  Value=64
  NOT : Logic  Operator=NOT  IconShape=distinctive  AllPortsSameDT=off  OutDataTypeStr=boolean
  Product{,1..6,8,16..23,35,142} (18 alike) : Product
  Switch_2 : Switch  Criteria=u2 ~= 0  OutDataTypeStr=fixdt(0,1,0)  SaturateOnIntegerOverflow=off  InputSameDT=off
  E_Y : Outport  LockScale=on
  wires:
  Constant/1 -> Product/2
  Y1/1 -> Product/1
  Constant1/1 -> Product1/2
  Y2/1 -> Product1/1
  Constant2/1 -> Product2/2
  Y3/1 -> Product2/1
  Constant6/1 -> Add/1
  Product/1 -> Add/2
  Product1/1 -> Add/3
  Product2/1 -> Add/4
  Add/1 -> Product6/1
  Add2/1 -> Product8/2, Product8/1
  Product4/1 -> Add/6
  Constant4/1 -> Product4/2
  Constant8/1 -> Product5/2
  Y6/1 -> Product5/1
  Product3/1 -> Add/5
  Y4/1 -> Product3/1
  Product5/1 -> Add/7
  Y5/1 -> Product4/1
  Constant3/1 -> Product3/2
  Product19/1 -> Add/11
  Constant20/1 -> Product21/2
  Constant18/1 -> Product19/2
  Product18/1 -> Add/10
  Constant15/1 -> Product16/2
  Constant16/1 -> Product17/2
  Y11/1 -> Product20/1
  Product20/1 -> Add/12
  Y8/1 -> Product17/1
  Y10/1 -> Product19/1
  Switch_2/1 -> Product16/1
  Constant19/1 -> Product20/2
  Product16/1 -> Add/8
  Y9/1 -> Product18/1
  Constant17/1 -> Product18/2
  Product21/1 -> Add/13
  Y12/1 -> Product21/1
  Product17/1 -> Add/9
  Y14/1 -> Product23/1
  Product22/1 -> Add/14
  Product23/1 -> Add/15
  Constant21/1 -> Product22/2
  Constant22/1 -> Product23/2
  [EN_Y] -> Switch_2/2
  Y7/1 -> NOT/1, Switch_2/3  "PBIT28"
  NOT/1 -> Switch_2/1
  Y13/1 -> Product22/1
  EN_Y/1 -> [EN_Y]
  shifted_coeff/1 -> [shifted_coeff]
  Product142/1 -> E_Y/1
  [shifted_coeff] -> Product142/2
  Product6/1 -> Add2/1
  Product8/1 -> Product142/1
  N/1 -> Add2/2
  X/1 -> Product6/2
  Y15/1 -> Product35/1
  Product35/1 -> Add/16
  Constant34/1 -> Product35/2

== system Model_with_decision_and_sieve/Y8 ==
  Y1 : Inport  OutDataTypeStr=fixdt(0,1,0)  LockScale=on
  Y2 : Inport  Port=2  OutDataTypeStr=fixdt(0,1,0)  LockScale=on
  Y3 : Inport  Port=3  OutDataTypeStr=fixdt(0,1,0)  LockScale=on
  Y4 : Inport  Port=4  OutDataTypeStr=fixdt(0,1,0)  LockScale=on
  Y5 : Inport  Port=5  OutDataTypeStr=fixdt(0,1,0)  LockScale=on
  Y6 : Inport  Port=6  OutDataTypeStr=fixdt(0,1,0)  LockScale=on
  Y7 : Inport  Port=7  OutDataTypeStr=fixdt(0,1,0)  LockScale=on
  Y8 : Inport  Port=8  OutDataTypeStr=fixdt(0,1,0)  LockScale=on
  Y9 : Inport  Port=9  OutDataTypeStr=fixdt(0,1,0)  LockScale=on
  Y10 : Inport  Port=10  OutDataTypeStr=fixdt(0,1,0)  LockScale=on
  Y11 : Inport  Port=11  OutDataTypeStr=fixdt(0,1,0)  LockScale=on
  Y12 : Inport  Port=12  OutDataTypeStr=fixdt(0,1,0)  LockScale=on
  Y13 : Inport  Port=13  OutDataTypeStr=fixdt(0,1,0)  LockScale=on
  Y14 : Inport  Port=14  OutDataTypeStr=fixdt(0,1,0)  LockScale=on
  Y15 : Inport  Port=15  OutDataTypeStr=fixdt(0,1,0)  LockScale=on
  X : Inport  Port=16
  N : Inport  Port=17  LockScale=on
  shifted_coeff : Inport  Port=18  LockScale=on
  EN_Y : Inport  Port=19  OutDataTypeStr=fixdt(0,1,0)  LockScale=on
  Add : Sum  Inputs=++++++++++++++++
  Add2 : Sum  Inputs=+-
  Constant : Constant  Value=2
  Constant1 : Constant  Value=4
  Constant15 : Constant  Value=128
  Constant16 : Constant  Value=256
  Constant17 : Constant  Value=512
  Constant18 : Constant  Value=1024
  Constant19 : Constant  Value=2048
  Constant2 : Constant  Value=8
  Constant20 : Constant  Value=4096
  Constant21 : Constant  Value=8192
  Constant22 : Constant  Value=16384
  Constant3 : Constant  Value=16
  Constant34 : Constant  Value=32768
  Constant4 : Constant  Value=32
  Constant6 : Constant
  Constant8 : Constant  Value=64
  NOT : Logic  Operator=NOT  IconShape=distinctive  AllPortsSameDT=off  OutDataTypeStr=boolean
  Product{,1..6,8,16..23,35,142} (18 alike) : Product
  Switch_2 : Switch  Criteria=u2 ~= 0  OutDataTypeStr=fixdt(0,1,0)  SaturateOnIntegerOverflow=off  InputSameDT=off
  E_Y : Outport  LockScale=on
  wires:
  Constant34/1 -> Product35/2
  Product35/1 -> Add/16
  Y15/1 -> Product35/1
  X/1 -> Product6/2
  N/1 -> Add2/2
  Product8/1 -> Product142/1
  Product6/1 -> Add2/1
  [shifted_coeff] -> Product142/2
  Product142/1 -> E_Y/1
  shifted_coeff/1 -> [shifted_coeff]
  EN_Y/1 -> [EN_Y]
  Y13/1 -> Product22/1
  NOT/1 -> Switch_2/1
  Y8/1 -> Switch_2/3, NOT/1  "PBIT28"
  [EN_Y] -> Switch_2/2
  Constant22/1 -> Product23/2
  Constant21/1 -> Product22/2
  Product23/1 -> Add/15
  Product22/1 -> Add/14
  Y14/1 -> Product23/1
  Product17/1 -> Add/9
  Y12/1 -> Product21/1
  Product21/1 -> Add/13
  Constant17/1 -> Product18/2
  Y9/1 -> Product18/1
  Product16/1 -> Add/8
  Constant19/1 -> Product20/2
  Y7/1 -> Product16/1
  Y10/1 -> Product19/1
  Switch_2/1 -> Product17/1
  Product20/1 -> Add/12
  Y11/1 -> Product20/1
  Constant16/1 -> Product17/2
  Constant15/1 -> Product16/2
  Product18/1 -> Add/10
  Constant18/1 -> Product19/2
  Constant20/1 -> Product21/2
  Product19/1 -> Add/11
  Constant3/1 -> Product3/2
  Y5/1 -> Product4/1
  Product5/1 -> Add/7
  Y4/1 -> Product3/1
  Product3/1 -> Add/5
  Y6/1 -> Product5/1
  Constant8/1 -> Product5/2
  Constant4/1 -> Product4/2
  Product4/1 -> Add/6
  Add2/1 -> Product8/1, Product8/2
  Add/1 -> Product6/1
  Product2/1 -> Add/4
  Product1/1 -> Add/3
  Product/1 -> Add/2
  Constant6/1 -> Add/1
  Y3/1 -> Product2/1
  Constant2/1 -> Product2/2
  Y2/1 -> Product1/1
  Constant1/1 -> Product1/2
  Y1/1 -> Product/1
  Constant/1 -> Product/2

== system Model_with_decision_and_sieve/Y9 ==
  Y1 : Inport  OutDataTypeStr=fixdt(0,1,0)  LockScale=on
  Y2 : Inport  Port=2  OutDataTypeStr=fixdt(0,1,0)  LockScale=on
  Y3 : Inport  Port=3  OutDataTypeStr=fixdt(0,1,0)  LockScale=on
  Y4 : Inport  Port=4  OutDataTypeStr=fixdt(0,1,0)  LockScale=on
  Y5 : Inport  Port=5  OutDataTypeStr=fixdt(0,1,0)  LockScale=on
  Y6 : Inport  Port=6  OutDataTypeStr=fixdt(0,1,0)  LockScale=on
  Y7 : Inport  Port=7  OutDataTypeStr=fixdt(0,1,0)  LockScale=on
  Y8 : Inport  Port=8  OutDataTypeStr=fixdt(0,1,0)  LockScale=on
  Y9 : Inport  Port=9  OutDataTypeStr=fixdt(0,1,0)  LockScale=on
  Y10 : Inport  Port=10  OutDataTypeStr=fixdt(0,1,0)  LockScale=on
  Y11 : Inport  Port=11  OutDataTypeStr=fixdt(0,1,0)  LockScale=on
  Y12 : Inport  Port=12  OutDataTypeStr=fixdt(0,1,0)  LockScale=on
  Y13 : Inport  Port=13  OutDataTypeStr=fixdt(0,1,0)  LockScale=on
  Y14 : Inport  Port=14  OutDataTypeStr=fixdt(0,1,0)  LockScale=on
  Y15 : Inport  Port=15  OutDataTypeStr=fixdt(0,1,0)  LockScale=on
  X : Inport  Port=16
  N : Inport  Port=17  LockScale=on
  shifted_coeff : Inport  Port=18  LockScale=on
  EN_Y : Inport  Port=19  OutDataTypeStr=fixdt(0,1,0)  LockScale=on
  Add : Sum  Inputs=++++++++++++++++
  Add2 : Sum  Inputs=+-
  Constant : Constant  Value=2
  Constant1 : Constant  Value=4
  Constant15 : Constant  Value=128
  Constant16 : Constant  Value=256
  Constant17 : Constant  Value=512
  Constant18 : Constant  Value=1024
  Constant19 : Constant  Value=2048
  Constant2 : Constant  Value=8
  Constant20 : Constant  Value=4096
  Constant21 : Constant  Value=8192
  Constant22 : Constant  Value=16384
  Constant3 : Constant  Value=16
  Constant34 : Constant  Value=32768
  Constant4 : Constant  Value=32
  Constant6 : Constant
  Constant8 : Constant  Value=64
  NOT : Logic  Operator=NOT  IconShape=distinctive  AllPortsSameDT=off  OutDataTypeStr=boolean
  Product{,1..6,8,16..23,35,142} (18 alike) : Product
  Switch_2 : Switch  Criteria=u2 ~= 0  OutDataTypeStr=fixdt(0,1,0)  SaturateOnIntegerOverflow=off  InputSameDT=off
  E_Y : Outport  LockScale=on
  wires:
  Constant/1 -> Product/2
  Y1/1 -> Product/1
  Constant1/1 -> Product1/2
  Y2/1 -> Product1/1
  Constant2/1 -> Product2/2
  Y3/1 -> Product2/1
  Constant6/1 -> Add/1
  Product/1 -> Add/2
  Product1/1 -> Add/3
  Product2/1 -> Add/4
  Add/1 -> Product6/1
  Add2/1 -> Product8/2, Product8/1
  Product4/1 -> Add/6
  Constant4/1 -> Product4/2
  Constant8/1 -> Product5/2
  Y6/1 -> Product5/1
  Product3/1 -> Add/5
  Y4/1 -> Product3/1
  Product5/1 -> Add/7
  Y5/1 -> Product4/1
  Constant3/1 -> Product3/2
  Product19/1 -> Add/11
  Constant20/1 -> Product21/2
  Constant18/1 -> Product19/2
  Product18/1 -> Add/10
  Constant15/1 -> Product16/2
  Constant16/1 -> Product17/2
  Y11/1 -> Product20/1
  Product20/1 -> Add/12
  Y8/1 -> Product17/1
  Y10/1 -> Product19/1
  Y7/1 -> Product16/1
  Constant19/1 -> Product20/2
  Product16/1 -> Add/8
  Switch_2/1 -> Product18/1
  Constant17/1 -> Product18/2
  Product21/1 -> Add/13
  Y12/1 -> Product21/1
  Product17/1 -> Add/9
  Y14/1 -> Product23/1
  Product22/1 -> Add/14
  Product23/1 -> Add/15
  Constant21/1 -> Product22/2
  Constant22/1 -> Product23/2
  [EN_Y] -> Switch_2/2
  Y9/1 -> Switch_2/3, NOT/1  "PBIT28"
  NOT/1 -> Switch_2/1
  Y13/1 -> Product22/1
  EN_Y/1 -> [EN_Y]
  shifted_coeff/1 -> [shifted_coeff]
  Product142/1 -> E_Y/1
  [shifted_coeff] -> Product142/2
  Product6/1 -> Add2/1
  Product8/1 -> Product142/1
  N/1 -> Add2/2
  X/1 -> Product6/2
  Y15/1 -> Product35/1
  Product35/1 -> Add/16
  Constant34/1 -> Product35/2

== system Model_with_decision_and_sieve/Modulo_X/EN=0 Block ==
  IN : Inport
  Action Port : ActionPort  ActionPortLabel=else
  Out1 : Outport
  wires:
  IN/1 -> Out1/1

== system Model_with_decision_and_sieve/Modulo_X/EN=1 Block ==
  N : Inport
  X_Sieve : Inport  Port=2
  Action Port : ActionPort  ActionPortLabel=if(u1 > 0)
  Constant127 : Constant
  Constant128 : Constant  Value=2
  Mod1 : Math  Operator=mod
  Subtract77 : Sum  Inputs=+-
  Switch1 : Switch  Criteria=u2 ~= 0  SaturateOnIntegerOverflow=off  InputSameDT=off
  OUT : Outport
  wires:
  Subtract77/1 -> Switch1/2
  Constant127/1 -> Subtract77/2
  X_Sieve/1 -> Switch1/1, Subtract77/1
  Switch1/1 -> Mod1/2
  Constant128/1 -> Switch1/3
  N/1 -> Mod1/1
  Mod1/1 -> OUT/1

== system Model_with_decision_and_sieve/Modulo_Y/EN=0 Block ==
  IN : Inport
  Action Port : ActionPort  ActionPortLabel=else
  Out1 : Outport
  wires:
  IN/1 -> Out1/1

== system Model_with_decision_and_sieve/Modulo_Y/EN=1 Block ==
  N : Inport
  Y_Sieve : Inport  Port=2
  Action Port : ActionPort  ActionPortLabel=if(u1 > 0)
  Constant127 : Constant
  Constant128 : Constant  Value=2
  Mod1 : Math  Operator=mod
  Subtract77 : Sum  Inputs=+-
  Switch1 : Switch  Criteria=u2 ~= 0  SaturateOnIntegerOverflow=off  InputSameDT=off
  OUT : Outport
  wires:
  Subtract77/1 -> Switch1/2
  Constant127/1 -> Subtract77/2
  Y_Sieve/1 -> Switch1/1, Subtract77/1
  Switch1/1 -> Mod1/2
  Constant128/1 -> Switch1/3
  N/1 -> Mod1/1
  Mod1/1 -> OUT/1

== system Model_with_decision_and_sieve/Pbit_1/EN=0 Block ==
  IN : Inport
  Action Port : ActionPort  ActionPortLabel=else
  Out1 : Outport
  wires:
  IN/1 -> Out1/1

== system Model_with_decision_and_sieve/Pbit_1/EN=1 Block ==
  note: this is boolean
  note: threshold is subtracted from the sum of total input and random value to implement > 1 comparison
  IN : Inport
  Action Port : ActionPort  ActionPortLabel=if(u1 > 0)
  Add : Sum
  Add1 : Sum
  Compare To Constant : simulink/Logic and Bit Operations/Compare To Constant  relop=>  const=1  OutDataTypeStr=boolean
  Constant : Constant  Value=-1
  Constant1 : Constant
  Constant2 : Constant
  Divide : Product  Inputs=*/
  Math Function : Math
  Product : Product
  Uniform Random Number : UniformRandomNumber  Minimum=0  Seed=s1  SampleTime=1
  OUT : Outport
  wires:
  Add1/1 -> Divide/2
  Constant2/1 -> Divide/1
  Math Function/1 -> Add1/1
  Product/1 -> Math Function/1
  Constant1/1 -> Add1/2
  Constant/1 -> Product/2
  Divide/1 -> Add/1
  IN/1 -> Product/1
  Compare To Constant/1 -> OUT/1
  Add/1 -> Compare To Constant/1
  Uniform Random Number/1 -> Add/2

== system Model_with_decision_and_sieve/Pbit_10/EN=0 Block ==
  IN : Inport
  Action Port : ActionPort  ActionPortLabel=else
  Out1 : Outport
  wires:
  IN/1 -> Out1/1

== system Model_with_decision_and_sieve/Pbit_10/EN=1 Block ==
  note: this is boolean
  note: threshold is subtracted from the sum of total input and random value to implement > 1 comparison
  IN : Inport
  Action Port : ActionPort  ActionPortLabel=if(u1 > 0)
  Add : Sum
  Add1 : Sum
  Compare To Constant : simulink/Logic and Bit Operations/Compare To Constant  relop=>  const=1  OutDataTypeStr=boolean
  Constant : Constant  Value=-1
  Constant1 : Constant
  Constant2 : Constant
  Divide : Product  Inputs=*/
  Math Function : Math
  Product : Product
  Uniform Random Number : UniformRandomNumber  Minimum=0  Seed=s10  SampleTime=1
  OUT : Outport
  wires:
  Add1/1 -> Divide/2
  Constant2/1 -> Divide/1
  Math Function/1 -> Add1/1
  Product/1 -> Math Function/1
  Constant1/1 -> Add1/2
  Constant/1 -> Product/2
  Divide/1 -> Add/1
  IN/1 -> Product/1
  Compare To Constant/1 -> OUT/1
  Add/1 -> Compare To Constant/1
  Uniform Random Number/1 -> Add/2

== system Model_with_decision_and_sieve/Pbit_11/EN=0 Block ==
  IN : Inport
  Action Port : ActionPort  ActionPortLabel=else
  Out1 : Outport
  wires:
  IN/1 -> Out1/1

== system Model_with_decision_and_sieve/Pbit_11/EN=1 Block ==
  note: this is boolean
  note: threshold is subtracted from the sum of total input and random value to implement > 1 comparison
  IN : Inport
  Action Port : ActionPort  ActionPortLabel=if(u1 > 0)
  Add : Sum
  Add1 : Sum
  Compare To Constant : simulink/Logic and Bit Operations/Compare To Constant  relop=>  const=1  OutDataTypeStr=boolean
  Constant : Constant  Value=-1
  Constant1 : Constant
  Constant2 : Constant
  Divide : Product  Inputs=*/
  Math Function : Math
  Product : Product
  Uniform Random Number : UniformRandomNumber  Minimum=0  Seed=s11  SampleTime=1
  OUT : Outport
  wires:
  Add1/1 -> Divide/2
  Constant2/1 -> Divide/1
  Math Function/1 -> Add1/1
  Product/1 -> Math Function/1
  Constant1/1 -> Add1/2
  Constant/1 -> Product/2
  Divide/1 -> Add/1
  IN/1 -> Product/1
  Compare To Constant/1 -> OUT/1
  Add/1 -> Compare To Constant/1
  Uniform Random Number/1 -> Add/2

== system Model_with_decision_and_sieve/Pbit_12/EN=0 Block ==
  IN : Inport
  Action Port : ActionPort  ActionPortLabel=else
  Out1 : Outport
  wires:
  IN/1 -> Out1/1

== system Model_with_decision_and_sieve/Pbit_12/EN=1 Block ==
  note: this is boolean
  note: threshold is subtracted from the sum of total input and random value to implement > 1 comparison
  IN : Inport
  Action Port : ActionPort  ActionPortLabel=if(u1 > 0)
  Add : Sum
  Add1 : Sum
  Compare To Constant : simulink/Logic and Bit Operations/Compare To Constant  relop=>  const=1  OutDataTypeStr=boolean
  Constant : Constant  Value=-1
  Constant1 : Constant
  Constant2 : Constant
  Divide : Product  Inputs=*/
  Math Function : Math
  Product : Product
  Uniform Random Number : UniformRandomNumber  Minimum=0  Seed=s12  SampleTime=1
  OUT : Outport
  wires:
  Add1/1 -> Divide/2
  Constant2/1 -> Divide/1
  Math Function/1 -> Add1/1
  Product/1 -> Math Function/1
  Constant1/1 -> Add1/2
  Constant/1 -> Product/2
  Divide/1 -> Add/1
  IN/1 -> Product/1
  Compare To Constant/1 -> OUT/1
  Add/1 -> Compare To Constant/1
  Uniform Random Number/1 -> Add/2

== system Model_with_decision_and_sieve/Pbit_13/EN=0 Block ==
  IN : Inport
  Action Port : ActionPort  ActionPortLabel=else
  Out1 : Outport
  wires:
  IN/1 -> Out1/1

== system Model_with_decision_and_sieve/Pbit_13/EN=1 Block ==
  note: threshold is subtracted from the sum of total input and random value to implement > 1 comparison
  note: this is boolean
  IN : Inport
  Action Port : ActionPort  ActionPortLabel=if(u1 > 0)
  Add : Sum
  Add1 : Sum
  Compare To Constant : simulink/Logic and Bit Operations/Compare To Constant  relop=>  const=1  OutDataTypeStr=boolean
  Constant : Constant  Value=-1
  Constant1 : Constant
  Constant2 : Constant
  Divide : Product  Inputs=*/
  Math Function : Math
  Product : Product
  Uniform Random Number : UniformRandomNumber  Minimum=0  Seed=s13  SampleTime=1
  OUT : Outport
  wires:
  Uniform Random Number/1 -> Add/2
  Add/1 -> Compare To Constant/1
  Compare To Constant/1 -> OUT/1
  IN/1 -> Product/1
  Divide/1 -> Add/1
  Constant/1 -> Product/2
  Constant1/1 -> Add1/2
  Product/1 -> Math Function/1
  Math Function/1 -> Add1/1
  Constant2/1 -> Divide/1
  Add1/1 -> Divide/2

== system Model_with_decision_and_sieve/Pbit_14/EN=0 Block ==
  IN : Inport
  Action Port : ActionPort  ActionPortLabel=else
  Out1 : Outport
  wires:
  IN/1 -> Out1/1

== system Model_with_decision_and_sieve/Pbit_14/EN=1 Block ==
  note: threshold is subtracted from the sum of total input and random value to implement > 1 comparison
  note: this is boolean
  IN : Inport
  Action Port : ActionPort  ActionPortLabel=if(u1 > 0)
  Add : Sum
  Add1 : Sum
  Compare To Constant : simulink/Logic and Bit Operations/Compare To Constant  relop=>  const=1  OutDataTypeStr=boolean
  Constant : Constant  Value=-1
  Constant1 : Constant
  Constant2 : Constant
  Divide : Product  Inputs=*/
  Math Function : Math
  Product : Product
  Uniform Random Number : UniformRandomNumber  Minimum=0  Seed=s14  SampleTime=1
  OUT : Outport
  wires:
  Uniform Random Number/1 -> Add/2
  Add/1 -> Compare To Constant/1
  Compare To Constant/1 -> OUT/1
  IN/1 -> Product/1
  Divide/1 -> Add/1
  Constant/1 -> Product/2
  Constant1/1 -> Add1/2
  Product/1 -> Math Function/1
  Math Function/1 -> Add1/1
  Constant2/1 -> Divide/1
  Add1/1 -> Divide/2

== system Model_with_decision_and_sieve/Pbit_15/EN=0 Block ==
  IN : Inport
  Action Port : ActionPort  ActionPortLabel=else
  Out1 : Outport
  wires:
  IN/1 -> Out1/1

== system Model_with_decision_and_sieve/Pbit_15/EN=1 Block ==
  note: this is boolean
  note: threshold is subtracted from the sum of total input and random value to implement > 1 comparison
  IN : Inport
  Action Port : ActionPort  ActionPortLabel=if(u1 > 0)
  Add : Sum
  Add1 : Sum
  Compare To Constant : simulink/Logic and Bit Operations/Compare To Constant  relop=>  const=1  OutDataTypeStr=boolean
  Constant : Constant  Value=-1
  Constant1 : Constant
  Constant2 : Constant
  Divide : Product  Inputs=*/
  Math Function : Math
  Product : Product
  Uniform Random Number : UniformRandomNumber  Minimum=0  Seed=s15  SampleTime=1
  OUT : Outport
  wires:
  Add1/1 -> Divide/2
  Constant2/1 -> Divide/1
  Math Function/1 -> Add1/1
  Product/1 -> Math Function/1
  Constant1/1 -> Add1/2
  Constant/1 -> Product/2
  Divide/1 -> Add/1
  IN/1 -> Product/1
  Compare To Constant/1 -> OUT/1
  Add/1 -> Compare To Constant/1
  Uniform Random Number/1 -> Add/2

== system Model_with_decision_and_sieve/Pbit_2/EN=0 Block ==
  IN : Inport
  Action Port : ActionPort  ActionPortLabel=else
  Out1 : Outport
  wires:
  IN/1 -> Out1/1
